simulink model "atrias_boom_nmSt_kinSw_v4"  (R2015a)
settings: Solver=ode23t  StartTime=0.0  StopTime=t_end  FixedStep=0.001  MaxStep=1e-3  RelTol=1e-3
InitFcn:
  | addpath('../common/')
  | colors
StartFcn:
  | tic
StopFcn:
  | %stopscript
values from neighbouring files (symbols this model uses):
  dt_a_dTrunk_boom = 5    [main_1_nmSt_kinSw.m]    (also in main_2_nmSt_kinSw_v2.m; main_3_nmSt_kinSw_v3.m; main_4_nmSt_kinSw_v4.m)
  dt_fade_boomCtrl = 2    [main_1_nmSt_kinSw.m]    (also in main_2_nmSt_kinSw_v2.m; main_3_nmSt_kinSw_v3.m; main_4_nmSt_kinSw_v4.m)
  initial_boom_yaw = 15*pi/180    (= 0.261799387799)    [main_2_nmSt_kinSw_v2.m]    (also in main_3_nmSt_kinSw_v3.m; main_4_nmSt_kinSw_v4.m)
  kd_boom_roll_Ctrl = 0    [main_1_nmSt_kinSw - Copy.m]    (also in main_1_nmSt_kinSw.m; main_2_nmSt_kinSw_v2.m; main_3_nmSt_kinSw_v3.m; main_4_nmSt_kinSw_v4.m)
  kd_boom_yaw_Ctrl = 0.1*kp_boom_yaw_Ctrl    (= 100000000)    [main_1_nmSt_kinSw - Copy.m]    (also in main_1_nmSt_kinSw.m = 1000000000; main_2_nmSt_kinSw_v2.m = 10000000; main_3_nmSt_kinSw_v3.m = 10000000; main_4_nmSt_kinSw_v4.m = 10000000)
  kd_motor = 0.90*2*sqrt(3.75*kp_motor)    [main_1_nmSt_kinSw - Copy.m]
  kinSw_alpha_start = 100*pi/180    (= 1.74532925199)    [main_1_nmSt_kinSw - Copy.m]    (also in main_1_nmSt_kinSw.m = 1.91986217719; main_2_nmSt_kinSw_v2.m = 1.83259571459; main_3_nmSt_kinSw_v3.m = 1.83259571459; main_4_nmSt_kinSw_v4.m = 1.83259571459)
  kinSw_alpha_tgt = 80*pi/180    (= 1.3962634016)    [main_1_nmSt_kinSw - Copy.m]    (also in main_1_nmSt_kinSw.m = 1.2217304764; main_2_nmSt_kinSw_v2.m = 1.2217304764; main_3_nmSt_kinSw_v3.m = 1.2217304764; main_4_nmSt_kinSw_v4.m = 1.2217304764)
  kinSw_t_start = 1.5    [main_1_nmSt_kinSw - Copy.m]    (also in main_1_nmSt_kinSw.m; main_2_nmSt_kinSw_v2.m = 0.5; main_3_nmSt_kinSw_v3.m = 0.5; main_4_nmSt_kinSw_v4.m = 0.5)
  kp_boom_roll_Ctrl = 0    [main_1_nmSt_kinSw - Copy.m]    (also in main_1_nmSt_kinSw.m; main_2_nmSt_kinSw_v2.m; main_3_nmSt_kinSw_v3.m; main_4_nmSt_kinSw_v4.m)
  kp_boom_yaw_Ctrl = 1e9    (= 1000000000)    [main_1_nmSt_kinSw - Copy.m]    (also in main_1_nmSt_kinSw.m = 10000000000; main_2_nmSt_kinSw_v2.m = 100000000; main_3_nmSt_kinSw_v3.m = 100000000; main_4_nmSt_kinSw_v4.m = 100000000)
  kp_motor = 3000    [main_1_nmSt_kinSw - Copy.m]
  max_back_bar_angle = 262.4*pi/180    (= 4.57974395723)    [main_1_nmSt_kinSw - Copy.m]
  max_front_bar_angle = 194.8*pi/180    (= 3.39990138288)    [main_1_nmSt_kinSw - Copy.m]
  min_back_bar_angle = 165.0*pi/180    (= 2.87979326579)    [main_1_nmSt_kinSw - Copy.m]
  min_front_bar_angle = 98.0*pi/180    (= 1.71042266695)    [main_1_nmSt_kinSw - Copy.m]
  poser_LLegAlp = (initial_l_leg_angle -pi/2)*180/pi    (= 105)    [main_2_nmSt_kinSw_v2.m]    (also in main_3_nmSt_kinSw_v3.m; main_4_nmSt_kinSw_v4.m)
  poser_LLegLen = initial_l_leg_length    (= 0.88)    [main_2_nmSt_kinSw_v2.m]    (also in main_3_nmSt_kinSw_v3.m; main_4_nmSt_kinSw_v4.m)
  poser_RLegAlp = (initial_r_leg_angle -pi/2)*180/pi    (= 75)    [main_2_nmSt_kinSw_v2.m]    (also in main_3_nmSt_kinSw_v3.m; main_4_nmSt_kinSw_v4.m)
  poser_RLegLen = initial_r_leg_length    (= 0.9)    [main_2_nmSt_kinSw_v2.m]    (also in main_3_nmSt_kinSw_v3.m; main_4_nmSt_kinSw_v4.m)
  tEnd_boomCtrl = t_end    (= 20)    [main_1_nmSt_kinSw - Copy.m]    (also in main_1_nmSt_kinSw.m = 3; main_2_nmSt_kinSw_v2.m = 7.5; main_3_nmSt_kinSw_v3.m = 7.5; main_4_nmSt_kinSw_v4.m = 7.5)
  tStart_boomCtrl = 1    [main_1_nmSt_kinSw - Copy.m]    (also in main_1_nmSt_kinSw.m = 0; main_2_nmSt_kinSw_v2.m = 0.5; main_3_nmSt_kinSw_v3.m = 0.5; main_4_nmSt_kinSw_v4.m = 0.5)
  tune_kinSw_alpha_start = kinSw_alpha_start*180/pi    (= 105)    [main_2_nmSt_kinSw_v2.m]    (also in main_3_nmSt_kinSw_v3.m; main_4_nmSt_kinSw_v4.m)
  tune_kinSw_alpha_tgt = kinSw_alpha_tgt*180/pi    (= 70)    [main_2_nmSt_kinSw_v2.m]    (also in main_3_nmSt_kinSw_v3.m; main_4_nmSt_kinSw_v4.m)
  tune_kinSw_gClr_tgt = kinSw_gClr    (= 0.15)    [main_4_nmSt_kinSw_v4.m]
  tune_kinSw_gH_tgt = kinSw_gH_tgt    (= -0.01)    [main_4_nmSt_kinSw_v4.m]
  tune_M1_G = St_FGain_VAS*FmaxVAS    [main_2_nmSt_kinSw_v2.m]    (also in main_3_nmSt_kinSw_v3.m; main_4_nmSt_kinSw_v4.m)
  tune_M3_0 = CtrlPar_theta0*180/pi    [main_2_nmSt_kinSw_v2.m]    (also in main_3_nmSt_kinSw_v3.m; main_4_nmSt_kinSw_v4.m)
  tune_M3_D = St_GainDTh_HFL    [main_2_nmSt_kinSw_v2.m]    (also in main_3_nmSt_kinSw_v3.m; main_4_nmSt_kinSw_v4.m)
  tune_M3_P = St_GainTh_HFL    [main_2_nmSt_kinSw_v2.m]    (also in main_3_nmSt_kinSw_v3.m; main_4_nmSt_kinSw_v4.m)
  tune_M4_G = 1    [main_3_nmSt_kinSw_v3.m]    (also in main_4_nmSt_kinSw_v4.m)
  v_dTrunk_boom = 1.3    [main_1_nmSt_kinSw.m]    (also in main_2_nmSt_kinSw_v2.m; main_3_nmSt_kinSw_v3.m; main_4_nmSt_kinSw_v4.m)
undefined symbols (not defined in the file or in its folder): A1_notch_f1, A2_notch_f1, A_lpf_dtau, A_lpf_velocity, ankle_stiffness, B1_lpf_dtau, B1_lpf_velocity, B1_notch_f1, B2_lpf_dtau, B2_lpf_velocity, B2_notch_f1, b_hmotor, b_leg_spring, b_rotor, base_color_d, boom_color_d, boom_mount_to_center_diagonal, breakaway_friction, c_jointstop, contactThr, coulomb_friction, d_com, delta_phi_max, delta_phi_max_buffer, delta_phi_max_dropoff, delta_phi_min, fblink_color_d, floor_color_d, FmaxBFSH, FmaxGLU, FmaxHAM, FmaxHFL, FmaxRF, FmaxVAS, foot_color_d, FPCtrlPar, friction_linear_zone, g, gain_nodes_sea_torque, HIP_MTR_MAX_CONT_TORQUE, HIP_MTR_MAX_TORQUE, hshaft_color_d, initial_boom_pitch, initial_boom_roll, initial_hip_roll, initial_winch_angle, j_motor, k_gn, k_gt, k_leg_spring, K_notch_f1, k_phi, k_sea, Kb_leg, kd_lateral, kd_shin_max, kd_shin_min, kd_splay_max, kd_splay_min, kd_thigh_max ... (+186)
libraries: sm_lib x210, nesl_utility x140, simulink x65, simulink_extras x32, fl_lib x16, mblibv1 x2, commnoisgen2 x1
(part 1 of 17)
settings Model: CovSFcnEnable=off  Creator=wmartin  LastModifiedBy=smsong
settings SolverCC: MaxOrder=2  MaxConsecutiveZCs=100  ZeroCrossAlgorithm=Adaptive  InsertRTBMode=Never (minimum delay)
settings DataIOCC: LimitDataPoints=off  SaveOutput=off  SignalLogging=off  DSMLogging=off  ReturnWorkspaceOutputs=on  OutputTimes=[0:1/30:45]
settings OptimizationCC: UseDivisionForNetSlopeComputation=UseDivisionForReciprocalsOfIntegersOnly  UseFloatMulNetSlope=on  EnhancedBackFolding=on  MemcpyThreshold=1024  EfficientFloat2IntCast=on  SimCompilerOptimization=on  AccelVerboseBuild=on
settings DebuggingCC: AlgebraicLoopMsg=none  UnconnectedInputMsg=none  UnconnectedOutputMsg=none  UnconnectedLineMsg=none  StateNameClashWarn=warning
settings ModelReferenceCC: UpdateModelReferenceTargets=IfOutOfDate
settings SFSimCC: SFSimOverflowDetection=off  SFSimEcho=off
settings RTWCC: BuildConfiguration=Faster Runs
settings GRTTargetCC: MatFileLogging=off  SupportNonFinite=off
settings ExplorerConfigSet: InternalSimMechanicsExplorerSettings="<ExplorerConfiguration><canonicalview>planar_xy</canonicalview><AnimationSetting><BasePlaybackSpeed>1.0</BasePlaybackSpeed><PlaybackSpeedFactor>0.125</PlaybackSpeedFactor></AnimationSetting><TilePanel><TileInfo><Tiles Columns=\"1\" Count=\"1\" Rows=\"1\"><Column Left=\"2\" Weight=\"1\"/><Column Left=\"1588\"/><Row Top=\"2\" Weight=\"1\"/><Row Top=\"952\"/><Tile Height=\"1\" Width=\"1\" X=\"0\" Y=\"0\"/></Tiles></TileInfo><SceneInfo><SceneViewer><BGColor><R>0.89803922176361084</R><G>0.89803922176361084</G><B>0.94901961088180542</B></BGColor><Camera><Position><X>0</X><Y>1.5296000242233276</Y><Z>-13.796973836269585</Z></Position><Center><X>0</X><Y>1.5296000242233276</Y><Z>0</Z></Center><Up><X>0</X><Y>1</Y><Z>0</Z></Up><Left>-3.2532129764556887</Left><Right>3.2532129764556887</Right><Bottom>-1.6375799953937531</Bottom><Top>1.6375799953937531</Top></Camera></SceneViewer></SceneInfo></TilePanel></ExplorerConfiguration>"

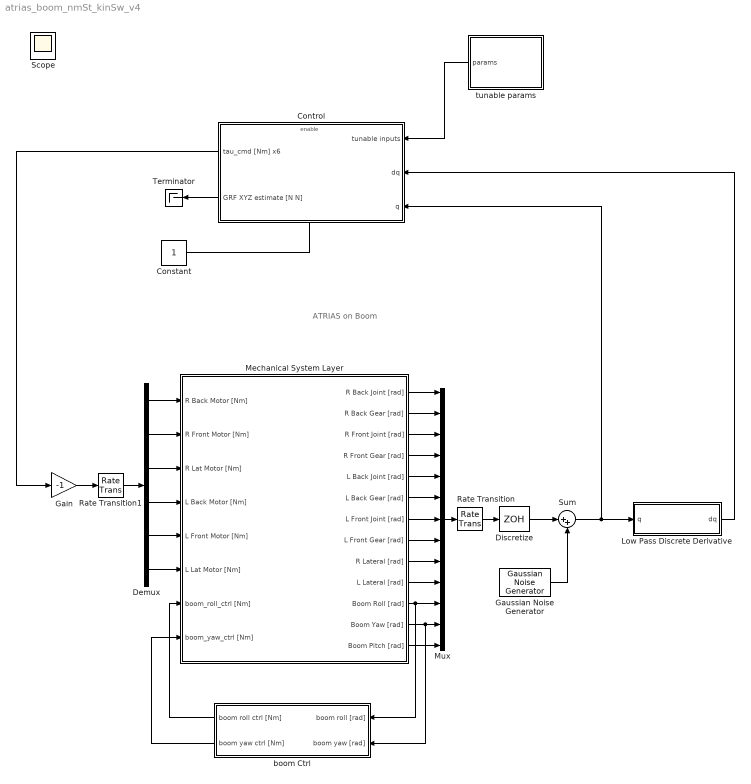
== system atrias_boom_nmSt_kinSw_v4 ==
  note: ATRIAS on Boom
  Constant : Constant
  Control : Subsystem
  Demux : Demux  Outputs=6
  Discretize : ZeroOrderHold  SampleTime=sample_time
  Gain : Gain  Gain=-1
  Gaussian Noise Generator : commnoisgen2/Gaussian Noise Generator  m=0  d=sensor_noise_variance  s=41  Ts=sample_time  frameBased=off  sampPerFrame=1  orient=off  outDataType=double
  Low Pass Discrete Derivative : Subsystem
  Mechanical System Layer : Subsystem
  Mux : Mux  Inputs=13
  Rate Transition : RateTransition  OutPortSampleTime=sample_time
  Rate Transition1 : RateTransition  OutPortSampleTime=sample_time
  Sum : Sum  Inputs=|++
  Terminator : Terminator
  boom Ctrl : Subsystem
  tunable params : Subsystem
  Scope : Scope
      settings: SaveName=ScopeData35
  wires:
  Mechanical System Layer/1(R Back Joint [rad]) -> Mux/1
  Mechanical System Layer/2(R Back Gear [rad]) -> Mux/2
  Mechanical System Layer/3(R Front Joint [rad]) -> Mux/3
  Mechanical System Layer/4(R Front Gear [rad]) -> Mux/4
  Mechanical System Layer/5(L Back Joint [rad]) -> Mux/5
  Mechanical System Layer/6(L Back Gear [rad]) -> Mux/6
  Mechanical System Layer/7(L Front Joint [rad]) -> Mux/7
  Mechanical System Layer/8(L Front Gear [rad]) -> Mux/8
  Mechanical System Layer/9(R Lateral [rad]) -> Mux/9
  Mechanical System Layer/10(L Lateral [rad]) -> Mux/10
  Mechanical System Layer/11(Boom Roll [rad]) -> boom Ctrl/1(boom roll [rad]), Mux/11
  Mechanical System Layer/12(Boom Yaw [rad]) -> boom Ctrl/2(boom yaw [rad]), Mux/12
  Mechanical System Layer/13(Boom Pitch [rad]) -> Mux/13
  Mux/1 -> Rate Transition/1
  Demux/1 -> Mechanical System Layer/1(R Back Motor [Nm])
  Demux/2 -> Mechanical System Layer/2(R Front Motor [Nm])
  Demux/3 -> Mechanical System Layer/3(R Lat Motor [Nm])
  Demux/4 -> Mechanical System Layer/4(L Back Motor [Nm])
  Demux/5 -> Mechanical System Layer/5(L Front Motor [Nm])
  Demux/6 -> Mechanical System Layer/6(L Lat Motor [Nm])
  Discretize/1 -> Sum/1
  Gaussian Noise Generator/1 -> Sum/2
  Rate Transition1/1 -> Demux/1
  Rate Transition/1 -> Discretize/1
  Low Pass Discrete Derivative/1(dq) -> Control/2(dq)
  Constant/1 -> Control/Enable
  Sum/1 -> Control/3(q), Low Pass Discrete Derivative/1(q)
  Control/2(GRF XYZ estimate [N N]) -> Terminator/1
  Control/1(tau_cmd [Nm] x6) -> Gain/1
  Gain/1 -> Rate Transition1/1
  boom Ctrl/2(boom yaw ctrl [Nm]) -> Mechanical System Layer/8(boom_yaw_ctrl [Nm])
  boom Ctrl/1(boom roll ctrl [Nm]) -> Mechanical System Layer/7(boom_roll_ctrl [Nm])
  tunable params/1(params) -> Control/1(tunable inputs)

== system atrias_boom_nmSt_kinSw_v4/Control ==
  tunable inputs : Inport
  dq : Inport  Port=2
  q : Inport  Port=3
  Enable : EnablePort  StatesWhenEnabling=reset  PropagateVarSize=During execution
  Actuator Control : Subsystem
  Behavior Control : Subsystem
  Tunable Control Parameters : Subsystem
  tau_cmd [Nm] x6 : Outport  InitialOutput=[0 0 0 0 0 0]
  GRF XYZ estimate [N N] : Outport  Port=2  InitialOutput=[0 0 0]
  wires:
  q/1 -> Actuator Control/4(q), Behavior Control/2(q [rad] x13)
  dq/1 -> Actuator Control/5(dq), Behavior Control/1(dq [rad/s] x13)
  Behavior Control/1(Motor Torque Command [Nm] x6) -> Actuator Control/1(Desired Torque [Nm] x6)
  Actuator Control/1(tau_cmd [Nm] x6) -> tau_cmd [Nm] x6/1
  Behavior Control/2(SEA Torque Velocity Command [Nm] x4) -> Actuator Control/2(Desired SEA Torque Velocity [Nm] x4)
  Behavior Control/3(Force / Position Control [1/0] x4) -> Actuator Control/3(Enable SEA Control [1/0] x4)
  Behavior Control/4(GRF XYZ estimates [N N N]) -> GRF XYZ estimate [N N]/1
  tunable inputs/1 -> Tunable Control Parameters/1(tunable inputs)

== system atrias_boom_nmSt_kinSw_v4/Low Pass Discrete Derivative ==
  q : Inport
  Gain1 : Gain  Gain=1/sample_time
  discrete difference : Subsystem
  two_pole_filter : DiscreteTransferFcn  Numerator=[A_lpf_velocity 0 0]  Denominator=[1 B1_lpf_velocity B2_lpf_velocity]  SampleTime=sample_time
  dq : Outport
  wires:
  q/1 -> discrete difference/1(in)
  two_pole_filter/1 -> dq/1
  Gain1/1 -> two_pole_filter/1
  discrete difference/1(out) -> Gain1/1

== system atrias_boom_nmSt_kinSw_v4/Mechanical System Layer ==
  R Back Motor [Nm] : Inport
  R Front Motor [Nm] : Inport  Port=2
  R Lat Motor [Nm] : Inport  Port=3
  L Back Motor [Nm] : Inport  Port=4
  L Front Motor [Nm] : Inport  Port=5
  L Lat Motor [Nm] : Inport  Port=6
  boom_roll_ctrl [Nm] : Inport  Port=7
  boom_yaw_ctrl [Nm] : Inport  Port=8
  Boom : Subsystem
      mask Display: image('../images/boom.png');
  Boom Base : Subsystem
      mask Display: image('../images/boom_base.png');
  Floor : Subsystem
  Floor Frame : sm_lib/Frames and Transforms/Rigid Transform  TranslationMethod=Cartesian  TranslationLengthUnit=m  TranslationStandardAxis=+Z  TranslationStandardOffset=0  TranslationCartesianOffset=[0 -0.03 0]  TranslationROffset=0  TranslationROffsetUnits=m  TranslationZOffset=0  TranslationZOffsetUnits=m  TranslationThetaOffset=0  TranslationThetaOffsetUnits=deg  RotationMethod=AlignedAxes  RotationAngleUnits=deg  RotationStandardAxis=+Z  RotationAngle=0  RotationArbitraryAxis=[0 0 1]  FollAlignAxisA=+Z  BaseAlignAxisA=+Y  FollAlignAxisB=+X  BaseAlignAxisB=+X  RotationMatrix=[1 0 0; 0 1 0; 0 0 1]  BlockFunction=simmechanics.library.frames_transforms.rigid_transform
  Ground : Subsystem
  Ground Contact Models : Subsystem
  L Hip Shaft : Subsystem
      mask Display: image(flipdim(imread('../images/hipshaft.JPG'),2));
  L Leg : Subsystem
      mask Display: image('../images/leg.JPG');
  Left Foot : Subsystem
      mask Display: image('../images/foot.png');
  Left Hip Roll Joint : Subsystem
  Pitch Joint : Subsystem
  R Hip Shaft : Subsystem
      mask Display: image('../images/hipshaft.JPG');
  R Leg : Subsystem
      mask Display: image('../images/leg.JPG');
  Right Foot : Subsystem
      mask Display: image('../images/foot.png');
  Right Hip Roll Joint : Subsystem
  Torso : Subsystem
      mask Display: image('../images/torso.png');
  Winch : Subsystem
  Yaw Joint : Subsystem
  Yaw Shaft : Subsystem
      mask Display: image('../images/boom_yaw_shaft.png');
  R Back Joint [rad] : Outport
  R Back Gear [rad] : Outport  Port=2
  R Front Joint [rad] : Outport  Port=3
  R Front Gear [rad] : Outport  Port=4
  L Back Joint [rad] : Outport  Port=5
  L Back Gear [rad] : Outport  Port=6
  L Front Joint [rad] : Outport  Port=7
  L Front Gear [rad] : Outport  Port=8
  R Lateral [rad] : Outport  Port=9
  L Lateral [rad] : Outport  Port=10
  Boom Roll [rad] : Outport  Port=11
  Boom Yaw [rad] : Outport  Port=12
  Boom Pitch [rad] : Outport  Port=13
  tag scope: qYaw=global
  wires:
  L Leg/1(Shin Joint [rad]) -> L Back Joint [rad]/1
  R Back Motor [Nm]/1 -> R Leg/1(Shin Motor [Nm])
  L Back Motor [Nm]/1 -> L Leg/1(Shin Motor [Nm])
  Right Hip Roll Joint/1(Hip Roll [rad]) -> R Lateral [rad]/1
  L Leg/3(Thigh Joint [rad]) -> L Front Joint [rad]/1
  Winch/1(Boom Roll [rad]) -> Boom Roll [rad]/1
  Left Hip Roll Joint/1(Hip Roll [rad]) -> L Lateral [rad]/1
  L Leg/4(Thigh Gear [rad]) -> L Front Gear [rad]/1
  R Leg/1(Shin Joint [rad]) -> R Back Joint [rad]/1
  R Leg/2(Shin Gear [rad]) -> R Back Gear [rad]/1
  L Leg/2(Shin Gear [rad]) -> L Back Gear [rad]/1
  R Leg/4(Thigh Gear [rad]) -> R Front Gear [rad]/1
  L Front Motor [Nm]/1 -> L Leg/2("Thigh Motor [Nm]  ")
  R Lat Motor [Nm]/1 -> Right Hip Roll Joint/1(Hip Motor [Nm])
  R Front Motor [Nm]/1 -> R Leg/2("Thigh Motor [Nm]  ")
  L Lat Motor [Nm]/1 -> Left Hip Roll Joint/1(Hip Motor [Nm])
  R Leg/3(Thigh Joint [rad]) -> R Front Joint [rad]/1
  Pitch Joint/1(Pitch [rad]) -> Boom Pitch [rad]/1
  Yaw Joint/1(Yaw [rad]) -> [qYaw], Boom Yaw [rad]/1
  boom_roll_ctrl [Nm]/1 -> Winch/1(boom_roll_ctrl [Nm])
  boom_yaw_ctrl [Nm]/1 -> Yaw Joint/1(boom_yaw_ctrl [Nm])
  connections:
  Torso/LConn1 -- Left Hip Roll Joint/RConn1
  Right Hip Roll Joint/RConn1 -- R Hip Shaft/RConn1
  Winch/RConn2 -- Yaw Shaft/RConn1
  Left Hip Roll Joint/LConn1 -- L Hip Shaft/LConn1
  Right Foot/LConn1 -- R Leg/LConn1
  R Leg/RConn1 -- R Hip Shaft/LConn1
  Torso/LConn2 -- Right Hip Roll Joint/LConn1
  L Leg/LConn1 -- L Hip Shaft/RConn1
  Left Foot/LConn1 -- L Leg/RConn1
  Pitch Joint/LConn1 -- Torso/RConn1
  Floor Frame/RConn1 -- Floor/LConn1
  Floor Frame/LConn1 -- Ground/RConn1 -- Boom Base/LConn1
  Boom/LConn1 -- Winch/RConn1
  Yaw Shaft/LConn1 -- Yaw Joint/RConn1
  Yaw Joint/LConn1 -- Boom Base/RConn1
  Pitch Joint/RConn1 -- Boom/RConn1
  Left Foot/RConn1 -- Ground Contact Models/RConn1
  Left Foot/RConn2 -- Ground Contact Models/RConn2
  Right Foot/RConn1 -- Ground Contact Models/RConn3
  Right Foot/RConn2 -- Ground Contact Models/RConn4

== system atrias_boom_nmSt_kinSw_v4/boom Ctrl ==
  boom roll [rad] : Inport
  boom yaw [rad] : Inport  Port=2
  Clock : Clock
  Constant1 : Constant  Value=tStart_boomCtrl
  Constant2 : Constant  Value=tEnd_boomCtrl
  Logical Operator : Logic  AllPortsSameDT=off  OutDataTypeStr=boolean
  Relational Operator : RelationalOperator  OutDataTypeStr=boolean
  Relational Operator1 : RelationalOperator  Operator=<=  OutDataTypeStr=boolean
  boom Ctrl : Subsystem
  boom roll ctrl [Nm] : Outport
  boom yaw ctrl [Nm] : Outport  Port=2
  wires:
  Relational Operator/1 -> Logical Operator/1
  Relational Operator1/1 -> Logical Operator/2
  Constant2/1 -> Relational Operator1/2
  boom yaw [rad]/1 -> boom Ctrl/2(Boom Yaw [rad])
  Constant1/1 -> Relational Operator/2
  boom roll [rad]/1 -> boom Ctrl/1(Boom Roll [rad])
  Logical Operator/1 -> boom Ctrl/Enable
  Clock/1 -> Relational Operator1/1, Relational Operator/1
  boom Ctrl/1(boom_roll_ctrl [Nm]) -> boom roll ctrl [Nm]/1  "roll"
  boom Ctrl/2(boom_yaw_ctrl [Nm]) -> boom yaw ctrl [Nm]/1  "yaw"

== system atrias_boom_nmSt_kinSw_v4/tunable params ==
  note: do not forget to set the params of the low pass filters!!
  Constant1 : Constant  Value=tune_M4_G
  Constant11 : Constant  Value=tune_M1_G
  Constant12 : Constant  Value=tune_M3_0
  Constant18 : Constant  Value=tune_M3_D
  Constant20 : Constant  Value=tune_M3_P
  Constant28 : Constant  Value=poser_RLegLen
  Constant29 : Constant  Value=poser_RLegAlp
  Constant30 : Constant  Value=poser_LLegLen
  Constant31 : Constant  Value=poser_LLegAlp
  Constant36 : Constant  Value=tune_kinSw_alpha_start
  Constant37 : Constant  Value=tune_kinSw_alpha_tgt
  Constant38 : Constant  Value=tune_kinSw_gH_tgt
  Constant39 : Constant  Value=tune_kinSw_gClr_tgt
  Mux2 : Mux  Inputs=13
  low pass filter : simulink_extras/Additional Linear/Transfer Fcn (with initial outputs)  N=[1]  D="[.5  1]"  Y0=tune_M1_G  U0=tune_M1_G
      settings: AttributesFormatString=pre-activation: %<Y0>
  low pass filter1 : simulink_extras/Additional Linear/Transfer Fcn (with initial outputs)  N=[1]  D="[.5  1]"  Y0=tune_M3_0  U0=tune_M3_0
      settings: AttributesFormatString=pre-activation: %<Y0>
  low pass filter10 : simulink_extras/Additional Linear/Transfer Fcn (with initial outputs)  N=[1]  D="[.5  1]"  Y0=poser_LLegLen  U0=poser_LLegLen
      settings: AttributesFormatString=pre-activation: %<Y0>
  low pass filter11 : simulink_extras/Additional Linear/Transfer Fcn (with initial outputs)  N=[1]  D="[.5  1]"  Y0=poser_LLegAlp  U0=poser_LLegAlp
      settings: AttributesFormatString=pre-activation: %<Y0>
  low pass filter12 : simulink_extras/Additional Linear/Transfer Fcn (with initial outputs)  N=[1]  D="[.5  1]"  Y0=tune_M4_G  U0=tune_M4_G
      settings: AttributesFormatString=pre-activation: %<Y0>
  low pass filter2 : simulink_extras/Additional Linear/Transfer Fcn (with initial outputs)  N=[1]  D="[.5  1]"  Y0=tune_M3_P  U0=tune_M3_P
      settings: AttributesFormatString=pre-activation: %<Y0>
  low pass filter3 : simulink_extras/Additional Linear/Transfer Fcn (with initial outputs)  N=[1]  D="[.5  1]"  Y0=tune_M3_D  U0=tune_M3_D
      settings: AttributesFormatString=pre-activation: %<Y0>
  low pass filter4 : simulink_extras/Additional Linear/Transfer Fcn (with initial outputs)  N=[1]  D="[.5  1]"  Y0=tune_kinSw_alpha_start  U0=tune_kinSw_alpha_start
      settings: AttributesFormatString=pre-activation: %<Y0>
  low pass filter5 : simulink_extras/Additional Linear/Transfer Fcn (with initial outputs)  N=[1]  D="[.5  1]"  Y0=tune_kinSw_alpha_tgt  U0=tune_kinSw_alpha_tgt
      settings: AttributesFormatString=pre-activation: %<Y0>
  low pass filter6 : simulink_extras/Additional Linear/Transfer Fcn (with initial outputs)  N=[1]  D="[.5  1]"  Y0=tune_kinSw_gH_tgt  U0=tune_kinSw_gH_tgt
      settings: AttributesFormatString=pre-activation: %<Y0>
  low pass filter7 : simulink_extras/Additional Linear/Transfer Fcn (with initial outputs)  N=[1]  D="[.5  1]"  Y0=tune_kinSw_gClr_tgt  U0=tune_kinSw_gClr_tgt
      settings: AttributesFormatString=pre-activation: %<Y0>
  low pass filter8 : simulink_extras/Additional Linear/Transfer Fcn (with initial outputs)  N=[1]  D="[.5  1]"  Y0=poser_RLegLen  U0=poser_RLegLen
      settings: AttributesFormatString=pre-activation: %<Y0>
  low pass filter9 : simulink_extras/Additional Linear/Transfer Fcn (with initial outputs)  N=[1]  D="[.5  1]"  Y0=poser_RLegAlp  U0=poser_RLegAlp
      settings: AttributesFormatString=pre-activation: %<Y0>
  params : Outport
  wires:
  Mux2/1 -> params/1
  Constant18/1 -> low pass filter3/1
  Constant11/1 -> low pass filter/1
  Constant36/1 -> low pass filter4/1
  Constant37/1 -> low pass filter5/1
  Constant12/1 -> low pass filter1/1
  Constant38/1 -> low pass filter6/1
  Constant39/1 -> low pass filter7/1
  Constant20/1 -> low pass filter2/1
  low pass filter/1 -> Mux2/1
  low pass filter1/1 -> Mux2/2
  low pass filter2/1 -> Mux2/3
  low pass filter3/1 -> Mux2/4
  low pass filter4/1 -> Mux2/6
  low pass filter5/1 -> Mux2/7
  low pass filter6/1 -> Mux2/8
  low pass filter7/1 -> Mux2/9
  Constant28/1 -> low pass filter8/1
  low pass filter8/1 -> Mux2/10
  Constant29/1 -> low pass filter9/1
  low pass filter9/1 -> Mux2/11
  Constant30/1 -> low pass filter10/1
  low pass filter10/1 -> Mux2/12
  Constant31/1 -> low pass filter11/1
  low pass filter11/1 -> Mux2/13
  Constant1/1 -> low pass filter12/1
  low pass filter12/1 -> Mux2/5

== system atrias_boom_nmSt_kinSw_v4/Control/Actuator Control ==
  note: Order:
      | backR
      | frontR
      | backL
      | frontL
  note: Motor Order:
      |
      | backR
      | frontR
      | latR
      | backL
      | frontL
      | latL
  Desired Torque [Nm] x6 : Inport  OutDataTypeStr=double  PortDimensions=6  SampleTime=sample_time
  Desired SEA Torque Velocity [Nm] x4 : Inport  Port=2  OutDataTypeStr=double  PortDimensions=4  SampleTime=sample_time
  Enable SEA Control [1/0] x4 : Inport  Port=3  OutDataTypeStr=boolean  PortDimensions=4  SampleTime=sample_time
  q : Inport  Port=4  OutDataTypeStr=double  PortDimensions=13  SampleTime=sample_time
  dq : Inport  Port=5  OutDataTypeStr=double  PortDimensions=13  SampleTime=sample_time
  Activate SEA Control : Subsystem
  Antiresonance Compensation : Subsystem
  Hip Motor Efficiency Compensation : Gain  Gain=1/lateral_motor_efficiency
  Leg Motor Efficiency Compensation : Gain  Gain=1/sagittal_motor_efficiency
  Mux{1..2,4..5} (4 alike) : Mux
  Mux3 : Mux  Inputs=2
  SEA Control Toggle : Subsystem
  SEA Controller (Torque) : Subsystem
  Selector12 : Selector  InputPortWidth=13  Indices=[5 6]
  Selector13 : Selector  InputPortWidth=13  Indices=[7 8]
  Selector15 : Selector  InputPortWidth=13  Indices=[1 2]
  Selector16 : Selector  InputPortWidth=13  Indices=[3 4]
  Selector{17..20,25..28} (8 alike) : Selector  InputPortWidth=2  Indices=[1]
  Selector2 : Selector  InputPortWidth=13  Indices=[5 6]
  Selector{21..24,29..32} (8 alike) : Selector  InputPortWidth=2  Indices=[2]
  Selector3 : Selector  InputPortWidth=6  Indices=[3 6]
  Selector33 : Selector  InputPortWidth=6  Indices=[1 2 4 5]
  Selector4 : Selector  InputPortWidth=13  Indices=[7 8]
  Selector6 : Selector  InputPortWidth=13  Indices=[1 2]
  Selector7 : Selector  InputPortWidth=13  Indices=[3 4]
  Selector8 : Selector  InputPortWidth=6  Indices=[1 2 5 3 4 6]
  Selector9 : Selector  InputPortWidth=6  Indices=[1 2 4 5]
  Terminator1 : Terminator
  Torque Limiter (outside) 1 : Saturate  UpperLimit=max_sagittal_unloaded_torque  LowerLimit=-max_sagittal_unloaded_torque
      settings: AttributesFormatString=Hi: %<UpperLimit>\nLo: %<LowerLimit>
  tau_desired_signals : Gain  Description=xPCTag(1)=tau_cmd_signal;
  tau_cmd [Nm] x6 : Outport  OutDataTypeStr=double  PortDimensions=6  SampleTime=0  InitialOutput=[0 0 0 0 0 0]
  wires:
  Selector3/1 -> Hip Motor Efficiency Compensation/1
  [dqFrontL] -> Selector32/1
  Selector29/1 -> Mux5/1
  Selector18/1 -> Mux1/2
  Selector19/1 -> Mux1/3
  Selector2/1 -> [qBackL]
  Selector15/1 -> [dqBackR]
  dq/1 -> Selector13/1, Selector15/1, Selector16/1, Selector12/1
  tau_desired_signals/1 -> Terminator1/1
  Selector7/1 -> [qFrontR]
  Torque Limiter (outside) 1/1 -> Activate SEA Control/3(Torque Signal [Nm] x4), SEA Control Toggle/3(tau_cmd)
  Desired Torque [Nm] x6/1 -> Selector33/1, Selector9/1, Selector3/1, tau_desired_signals/1
  Selector8/1 -> tau_cmd [Nm] x6/1
  Selector6/1 -> [qBackR]
  SEA Controller (Torque)/1(tau_cmd sagittal [Nm] x4) -> Activate SEA Control/1(SEA Control Signal [Nm] x4)
  SEA Controller (Torque)/2(tau_measured [Nm] x4) -> SEA Control Toggle/2(tau_measured)
  Activate SEA Control/1(Torque Command [Nm] x4) -> Leg Motor Efficiency Compensation/1
  q/1 -> Selector2/1, Selector7/1, Selector6/1, Selector4/1
  Selector16/1 -> [dqFrontR]
  Selector4/1 -> [qFrontL]
  Selector9/1 -> Antiresonance Compensation/1(Torque)
  [qBackL] -> Selector23/1
  Selector26/1 -> Mux4/2
  Selector30/1 -> Mux5/2
  Mux5/1 -> SEA Controller (Torque)/6(dphi_gear [rad/s] x4)
  Leg Motor Efficiency Compensation/1 -> Mux3/1
  Selector24/1 -> Mux2/4
  [qFrontR] -> Selector18/1
  [qFrontL] -> Selector20/1
  [qBackR] -> Selector21/1
  Antiresonance Compensation/1(Filtered Torque) -> Torque Limiter (outside) 1/1
  Selector13/1 -> [dqFrontL]
  Selector23/1 -> Mux2/3
  Mux1/1 -> SEA Controller (Torque)/1(phi_load [rad] x4)
  [dqFrontL] -> Selector28/1
  Desired SEA Torque Velocity [Nm] x4/1 -> SEA Controller (Torque)/4(dtau_des sagittal [Nm] x4)
  Selector25/1 -> Mux4/1
  Selector31/1 -> Mux5/3
  [dqBackL] -> Selector31/1
  Hip Motor Efficiency Compensation/1 -> Mux3/2
  Selector28/1 -> Mux4/4
  [qFrontL] -> Selector24/1
  Selector22/1 -> Mux2/2
  [dqFrontR] -> Selector30/1
  Selector32/1 -> Mux5/4
  Mux4/1 -> SEA Controller (Torque)/5(dphi_load [rad/s] x4)
  Mux3/1 -> Selector8/1
  [dqBackR] -> Selector29/1
  Selector27/1 -> Mux4/3
  [qFrontR] -> Selector22/1
  Selector21/1 -> Mux2/1
  [dqBackL] -> Selector27/1
  [dqBackR] -> Selector25/1
  Selector20/1 -> Mux1/4
  Selector17/1 -> Mux1/1
  [qBackR] -> Selector17/1
  [qBackL] -> Selector19/1
  Selector12/1 -> [dqBackL]
  Mux2/1 -> SEA Controller (Torque)/2(phi_gear [rad] x4)
  SEA Control Toggle/1(SEA Control on/off [1/0]) -> Activate SEA Control/2("SEA on/off [1/0] x4 ")
  Selector33/1 -> SEA Controller (Torque)/3(tau_des sagittal [Nm] x4)
  Enable SEA Control [1/0] x4/1 -> SEA Control Toggle/1(enable)
  [dqFrontR] -> Selector26/1

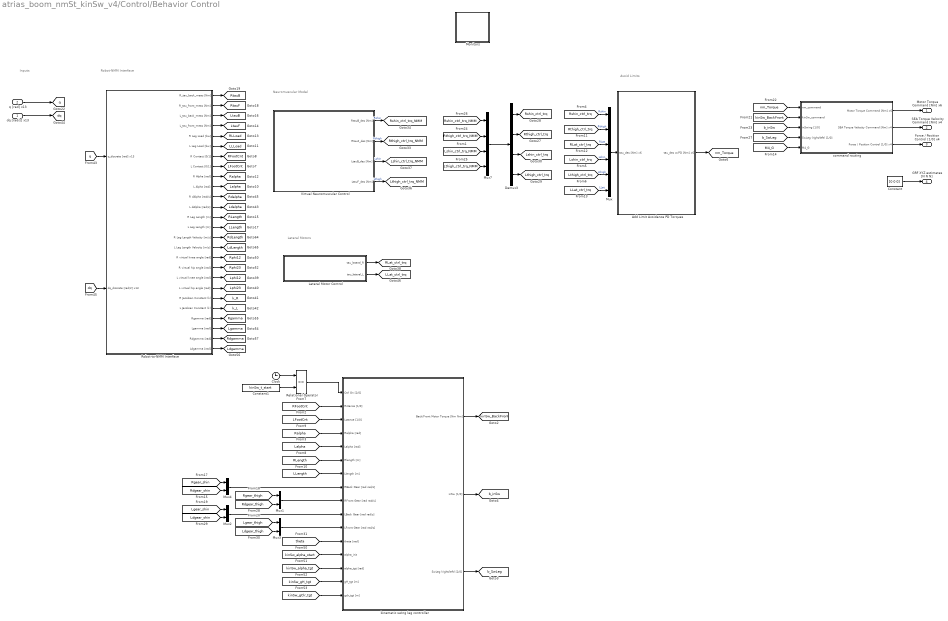
== system atrias_boom_nmSt_kinSw_v4/Control/Behavior Control ==
  note: Robot-NMM Interface
  note: Inputs
  note: Neuromuscular Model
  note: Avoid Limits
  note: Lateral Motors
  dq [rad/s] x13 : Inport
  q [rad] x13 : Inport  Port=2
  Add Limit Avoidance PD Torques : Subsystem
  Clock : Clock
  Constant : Constant  Value=[0 0 0]
  Constant1 : Constant  Value=kinSw_t_start
  Demux3 : Demux
  Lateral Motor Control : Subsystem
  Monitors : Subsystem
  Mux : Mux  Inputs=6
  Mux{1..4} (4 alike) : Mux  Inputs=2
  Mux7 : Mux
  Relational Operator : RelationalOperator
  Robot-to-NMM Interface : Subsystem
  Virtual Neuromuscular Control : Subsystem  SystemSampleTime=sample_time
  command routing : Subsystem
  kinematic swing leg controller : Subsystem
  Motor Torque Command [Nm] x6 : Outport  OutputWhenDisabled=reset  InitialOutput=[0 0 0 0 0 0]
  SEA Torque Velocity Command [Nm] x4 : Outport  Port=2  OutputWhenDisabled=reset  InitialOutput=[0 0 0 0 0 0]
  Force / Position Control [1/0] x4 : Outport  Port=3  OutputWhenDisabled=reset  InitialOutput=[0 0 0 0 0 0]
  GRF XYZ estimates [N N N] : Outport  Port=4  OutputWhenDisabled=reset  InitialOutput=[0 0 0 0 0 0]
  tag scope: LFootCnt=global, LLLoad=global, LLat_ctrl_trq=global, LLength=global, Lalpha=global, LdLength=global, Ldalpha=global, Ldgamma=global, Lgamma=global, Lphi12=global, Lphi23=global, Lshin_ctrl_trq=global, Lshin_ctrl_trq_NMM=global, LtauB=global, LtauF=global, Lthigh_ctrl_trq=global, Lthigh_ctrl_trq_NMM=global, RFootCnt=global, RLLoad=global, RLat_ctrl_trq=global, RLength=global, Ralpha=global, RdLength=global, Rdalpha=global, Rdgamma=global, Rgamma=global, Rphi12=global, Rphi23=global, Rshin_ctrl_trq=global, Rshin_ctrl_trq_NMM=global, RtauB=global, RtauF=global, Rthigh_ctrl_trq=global, Rthigh_ctrl_trq_NMM=global, b_SwLeg=global, b_inSw=global, dq=global, k_L=global, k_R=global, kinSw_BackFront=global, nm_Torque=global, q=global
  wires:
  [q] -> Robot-to-NMM Interface/1(q_discrete [rad] x13)
  [dq] -> Robot-to-NMM Interface/2(dq_discrete [rad/2] x13)
  Robot-to-NMM Interface/6(L Leg Load [bw]) -> [LLLoad]
  Robot-to-NMM Interface/5(R Leg Load [bw]) -> [RLLoad]
  Robot-to-NMM Interface/10(L Alpha [rad]) -> [Lalpha]
  Robot-to-NMM Interface/9(R Alpha [rad]) -> [Ralpha]
  Robot-to-NMM Interface/14(L Leg Length [m]) -> [LLength]
  Robot-to-NMM Interface/13(R Leg Length [m]) -> [RLength]
  Robot-to-NMM Interface/7(R Contact [0/1]) -> [RFootCnt]
  Robot-to-NMM Interface/8(L Contact [0/1]) -> [LFootCnt]
  Robot-to-NMM Interface/4(L_tau_front_meas [Nm]) -> [LtauF]
  Robot-to-NMM Interface/3(L_tau_back_meas [Nm]) -> [LtauB]
  Robot-to-NMM Interface/2(R_tau_front_meas [Nm]) -> [RtauF]
  Robot-to-NMM Interface/1(R_tau_back_meas [Nm]) -> [RtauB]
  Robot-to-NMM Interface/17(R virtual knee angle [rad]) -> [Rphi12]
  Robot-to-NMM Interface/18(R virtual hip angle [rad]) -> [Rphi23]
  Robot-to-NMM Interface/19(L virtual knee angle [rad]) -> [Lphi12]
  Robot-to-NMM Interface/20(L virtual hip angle [rad]) -> [Lphi23]
  Robot-to-NMM Interface/22(L Jacobian Constant (k)) -> [k_L]
  Robot-to-NMM Interface/21(R Jacobian Constant (k)) -> [k_R]
  Robot-to-NMM Interface/11(R dAlpha [rad/s]) -> [Rdalpha]
  Robot-to-NMM Interface/12(L dAlpha [rad/s]) -> [Ldalpha]
  Robot-to-NMM Interface/23(Rgamma [rad]) -> [Rgamma]
  Robot-to-NMM Interface/24(Lgamma [rad]) -> [Lgamma]
  Robot-to-NMM Interface/25(Rdgamma [rad]) -> [Rdgamma]
  Robot-to-NMM Interface/26(Ldgamma [rad]) -> [Ldgamma]
  Robot-to-NMM Interface/15(R Leg Length Velocity [m/s]) -> [RdLength]
  Robot-to-NMM Interface/16(L Leg Length Velocity [m/s]) -> [LdLength]
  Virtual Neuromuscular Control/1(RtauB_des [Nm]) -> [Rshin_ctrl_trq_NMM]  "Rshin"
  Virtual Neuromuscular Control/2(RtauF_des [Nm]) -> [Rthigh_ctrl_trq_NMM]  "Rthigh"
  Virtual Neuromuscular Control/3(LtauB_des [Nm]) -> [Lshin_ctrl_trq_NMM]  "Lshin"
  [Rshin_ctrl_trq_NMM] -> Mux7/1
  [Rthigh_ctrl_trq_NMM] -> Mux7/2
  [Lshin_ctrl_trq_NMM] -> Mux7/3
  [Lthigh_ctrl_trq_NMM] -> Mux7/4
  Demux3/4 -> [Lthigh_ctrl_trq]
  Demux3/3 -> [Lshin_ctrl_trq]
  Demux3/2 -> [Rthigh_ctrl_trq]
  Demux3/1 -> [Rshin_ctrl_trq]
  [Rshin_ctrl_trq] -> Mux/1  "Rshin"
  [Rthigh_ctrl_trq] -> Mux/2  "Rthigh"
  [RLat_ctrl_trq] -> Mux/3  "RLat"
  [Lshin_ctrl_trq] -> Mux/4  "Lshin"
  [Lthigh_ctrl_trq] -> Mux/5  "Lthigh"
  [LLat_ctrl_trq] -> Mux/6  "LLat"
  Mux/1 -> Add Limit Avoidance PD Torques/1(tau_des [Nm] x6)
  Lateral Motor Control/2(tau_lateral_L) -> [LLat_ctrl_trq]
  Lateral Motor Control/1(tau_lateral_R) -> [RLat_ctrl_trq]
  Constant/1 -> GRF XYZ estimates [N N N]/1
  q [rad] x13/1 -> [q]
  dq [rad/s] x13/1 -> [dq]
  Virtual Neuromuscular Control/4(LtauF_des [Nm]) -> [Lthigh_ctrl_trq_NMM]  "Lthigh"
  Mux7/1 -> Demux3/1
  [Ralpha] -> kinematic swing leg controller/4(Ralpha [rad])
  [Lalpha] -> kinematic swing leg controller/5(Lalpha [rad])
  [RFootCnt] -> kinematic swing leg controller/2(Rstance [1/0])
  [LFootCnt] -> kinematic swing leg controller/3(Lstance [1/0])
  [RLength] -> kinematic swing leg controller/6(Rlength [m])
  [LLength] -> kinematic swing leg controller/7(Llength [m])
  kinematic swing leg controller/1(Back/Front Motor Torque [Nm Nm]) -> [kinSw_BackFront]
  kinematic swing leg controller/3(SwLeg (right/left) [1/0]) -> [b_SwLeg]
  kinematic swing leg controller/2(inSw [1/0]) -> [b_inSw]
  Add Limit Avoidance PD Torques/1(tau_des w/PD [Nm] x6) -> [nm_Torque]
  [kinSw_BackFront] -> command routing/2(kinSw_command)
  [nm_Torque] -> command routing/1(nm_command)
  [b_inSw] -> command routing/3(inSwing [1/0])
  [b_SwLeg] -> command routing/4(SwLeg (right/left) [1/0])
  command routing/3(Force / Position Control [1/0] x4) -> Force / Position Control [1/0] x4/1
  [Rdgear_shin] -> Mux4/2
  [Rdgear_thigh] -> Mux1/2
  [Rgear_shin] -> Mux4/1
  [Rgear_thigh] -> Mux1/1
  [Lgear_shin] -> Mux2/1
  [Ldgear_shin] -> Mux2/2
  [Lgear_thigh] -> Mux3/1
  [Ldgear_thigh] -> Mux3/2
  Mux1/1 -> kinematic swing leg controller/9(RFront Gear [rad rad/s])
  Mux4/1 -> kinematic swing leg controller/8(RBack Gear [rad rad/s])
  Mux2/1 -> kinematic swing leg controller/10(LBack Gear [rad rad/s])
  Mux3/1 -> kinematic swing leg controller/11(LFront Gear [rad rad/s])
  command routing/1(Motor Torque Command [Nm] x6) -> Motor Torque Command [Nm] x6/1
  command routing/2(SEA Torque Velocity Command [Nm] x4) -> SEA Torque Velocity Command [Nm] x4/1
  Clock/1 -> Relational Operator/1
  Constant1/1 -> Relational Operator/2
  Relational Operator/1 -> kinematic swing leg controller/1(Ctrl On [1/0])
  [theta] -> kinematic swing leg controller/12(theta [rad])
  [kinSw_alpha_start] -> kinematic swing leg controller/13(alpha_init)
  [kinSw_alpha_tgt] -> kinematic swing leg controller/14(alpha_tgt [rad])
  [M4_G] -> command routing/5(M4_G)
  [kinSw_gH_tgt] -> kinematic swing leg controller/15(gH_tgt [m])
  [kinSw_gClr_tgt] -> kinematic swing leg controller/16(gclr_tgt [m])

== system atrias_boom_nmSt_kinSw_v4/Control/Tunable Control Parameters ==
  note: main controller
  note: intial poser
  tunable inputs : Inport
  Constant1 : Constant  Value=St_PreSHFL
  Constant10 : Constant  Value=TrCtrlPar
  Constant13 : Constant  Value=St_loffBFSH_VAS
  Constant14 : Constant  Value=St_LGainBFSH_VAS
  Constant15 : Constant  Value=St_loffBFSH
  Constant16 : Constant  Value=St_LGain_BFSH
  Constant17 : Constant  Value=St_SGainCGLU_HFL
  Constant19 : Constant  Value=St_SGainCHAM_HFL
  Constant2 : Constant  Value=LLCtrlPar
  Constant21 : Constant  Value=St_SGainGLU_HAM
  Constant22 : Constant  Value=St_SGainCHFL_GLU
  Constant23 : Constant  Value=St_SGainCRF_GLU
  Constant24 : Constant  Value=pi/2
  Constant3 : Constant  Value=St_PreSGLU
  Constant4 : Constant  Value=St_PreSHAM
  Constant5 : Constant  Value=St_PreSRF
  Constant6 : Constant  Value=FPCtrlPar
  Constant7 : Constant  Value=St_PreSVAS
  Constant8 : Constant  Value=St_PreSBFSH
  Constant9 : Constant  Value=SwCtrlPar
  Demux1 : Demux  Outputs=13
  Gain : Gain  Gain=1/FmaxVAS
  Gain{1..5} (5 alike) : Gain  Gain=pi/180
  Mux : Mux  Inputs=21
  Sum : Sum  Inputs=|++
  Sum1 : Sum  Inputs=|++
  tag scope: FPCtrlPar=global, LLCtrlPar=global, M4_G=global, StCtrlPar=global, SwCtrlPar=global, TrCtrlPar=global, kinSw_alpha_start=global, kinSw_alpha_tgt=global, kinSw_gClr_tgt=global, kinSw_gH_tgt=global, poser_LLegAng=global, poser_LLegLen=global, poser_RLegAng=global, poser_RLegLen=global, theta0=global
  wires:
  Constant6/1 -> [FPCtrlPar]
  Constant10/1 -> [TrCtrlPar]
  Constant9/1 -> [SwCtrlPar]
  Constant2/1 -> [LLCtrlPar]
  [tune_M3_0] -> Gain1/1
  [tune_M1_G] -> Gain/1
  Mux/1 -> [StCtrlPar]
  Gain1/1 -> [theta0]
  [poser_RLegLen] -> [poser_RLegLen]
  Sum/1 -> [poser_RLegAng]
  [poser_LLegLen] -> [poser_LLegLen]
  Sum1/1 -> [poser_LLegAng]
  [tune_kinSw_alpha_start] -> Gain4/1
  [tune_kinSw_alpha_tgt] -> Gain5/1
  Gain4/1 -> [kinSw_alpha_start]
  Gain5/1 -> [kinSw_alpha_tgt]
  [tune_kinSw_gH_tgt] -> [kinSw_gH_tgt]
  [tune_kinSw_gClr_tgt] -> [kinSw_gClr_tgt]
  [poser_RLegAlp] -> Gain3/1
  [poser_LLegAlp] -> Gain2/1
  Gain2/1 -> Sum1/1
  Gain3/1 -> Sum/1
  Constant24/1 -> Sum/2, Sum1/2
  Constant1/1 -> Mux/1
  Constant3/1 -> Mux/2
  Constant4/1 -> Mux/3
  Constant5/1 -> Mux/4
  Constant7/1 -> Mux/5
  Constant8/1 -> Mux/6
  Gain/1 -> Mux/7
  Constant13/1 -> Mux/8
  Constant14/1 -> Mux/9
  Constant15/1 -> Mux/10
  Constant16/1 -> Mux/11
  [tune_M3_P] -> Mux/14, Mux/12
  [tune_M3_D] -> Mux/15, Mux/13
  Constant21/1 -> Mux/21, Mux/16
  Constant17/1 -> Mux/17
  Constant19/1 -> Mux/18
  Constant22/1 -> Mux/19
  Constant23/1 -> Mux/20
  Demux1/1 -> [tune_M1_G]
  Demux1/2 -> [tune_M3_0]
  Demux1/3 -> [tune_M3_P]
  Demux1/4 -> [tune_M3_D]
  Demux1/6 -> [tune_kinSw_alpha_start]
  Demux1/7 -> [tune_kinSw_alpha_tgt]
  Demux1/8 -> [tune_kinSw_gH_tgt]
  Demux1/9 -> [tune_kinSw_gClr_tgt]
  Demux1/12 -> [poser_LLegLen]
  Demux1/13 -> [poser_LLegAlp]
  Demux1/10 -> [poser_RLegLen]
  Demux1/11 -> [poser_RLegAlp]
  Demux1/5 -> [tune_M4_G]
  tunable inputs/1 -> Demux1/1
  [tune_M4_G] -> [M4_G]

== system atrias_boom_nmSt_kinSw_v4/Low Pass Discrete Derivative/discrete difference ==
  note: q Order:
      |
      | backJointR
      | backGearR
      | frontJointR
      | frontGearR
      |
      | backJointL
      | backGearL
      | frontJointL
      | frontGearL
      |
      | latR
      | latL
      |
      | boomRoll
      | boomYaw
      | boomPitch
  in : Inport
  Demux : Demux  Outputs=13
  Mux : Mux  Inputs=13
  difference : simulink/Discrete/Difference  ICPrevInput=shin_initial_r  InputProcessing=Columns as channels (frame based)  OutMin=[]  OutMax=[]  OutDataType=fixdt(1, 16)  OutScaling=2^-10  DoSatur=off
  difference1 : simulink/Discrete/Difference  ICPrevInput=shin_initial_r  InputProcessing=Columns as channels (frame based)  OutMin=[]  OutMax=[]  OutDataType=fixdt(1, 16)  OutScaling=2^-10  DoSatur=off
  difference10 : simulink/Discrete/Difference  ICPrevInput=initial_boom_roll  InputProcessing=Columns as channels (frame based)  OutMin=[]  OutMax=[]  OutDataType=fixdt(1, 16)  OutScaling=2^-10  DoSatur=off
  difference11 : simulink/Discrete/Difference  ICPrevInput=initial_boom_yaw  InputProcessing=Columns as channels (frame based)  OutMin=[]  OutMax=[]  OutDataType=fixdt(1, 16)  OutScaling=2^-10  DoSatur=off
  difference12 : simulink/Discrete/Difference  ICPrevInput=initial_boom_pitch  InputProcessing=Columns as channels (frame based)  OutMin=[]  OutMax=[]  OutDataType=fixdt(1, 16)  OutScaling=2^-10  DoSatur=off
  difference2 : simulink/Discrete/Difference  ICPrevInput=thigh_initial_r  InputProcessing=Columns as channels (frame based)  OutMin=[]  OutMax=[]  OutDataType=fixdt(1, 16)  OutScaling=2^-10  DoSatur=off
  difference3 : simulink/Discrete/Difference  ICPrevInput=thigh_initial_r  InputProcessing=Columns as channels (frame based)  OutMin=[]  OutMax=[]  OutDataType=fixdt(1, 16)  OutScaling=2^-10  DoSatur=off
  difference4 : simulink/Discrete/Difference  ICPrevInput=shin_initial_l  InputProcessing=Columns as channels (frame based)  OutMin=[]  OutMax=[]  OutDataType=fixdt(1, 16)  OutScaling=2^-10  DoSatur=off
  difference5 : simulink/Discrete/Difference  ICPrevInput=shin_initial_l  InputProcessing=Columns as channels (frame based)  OutMin=[]  OutMax=[]  OutDataType=fixdt(1, 16)  OutScaling=2^-10  DoSatur=off
  difference6 : simulink/Discrete/Difference  ICPrevInput=thigh_initial_l  InputProcessing=Columns as channels (frame based)  OutMin=[]  OutMax=[]  OutDataType=fixdt(1, 16)  OutScaling=2^-10  DoSatur=off
  difference7 : simulink/Discrete/Difference  ICPrevInput=thigh_initial_l  InputProcessing=Columns as channels (frame based)  OutMin=[]  OutMax=[]  OutDataType=fixdt(1, 16)  OutScaling=2^-10  DoSatur=off
  difference8 : simulink/Discrete/Difference  ICPrevInput=initial_hip_roll  InputProcessing=Columns as channels (frame based)  OutMin=[]  OutMax=[]  OutDataType=fixdt(1, 16)  OutScaling=2^-10  DoSatur=off
  difference9 : simulink/Discrete/Difference  ICPrevInput=initial_hip_roll  InputProcessing=Columns as channels (frame based)  OutMin=[]  OutMax=[]  OutDataType=fixdt(1, 16)  OutScaling=2^-10  DoSatur=off
  out : Outport
  wires:
  Demux/1 -> difference/1
  in/1 -> Demux/1
  Mux/1 -> out/1
  Demux/2 -> difference1/1
  difference1/1 -> Mux/2
  Demux/3 -> difference2/1
  difference2/1 -> Mux/3
  Demux/4 -> difference3/1
  difference3/1 -> Mux/4
  Demux/5 -> difference4/1
  difference4/1 -> Mux/5
  Demux/6 -> difference5/1
  difference5/1 -> Mux/6
  Demux/7 -> difference6/1
  difference6/1 -> Mux/7
  Demux/8 -> difference7/1
  difference7/1 -> Mux/8
  Demux/9 -> difference8/1
  difference8/1 -> Mux/9
  Demux/10 -> difference9/1
  difference9/1 -> Mux/10
  Demux/11 -> difference10/1
  difference10/1 -> Mux/11
  Demux/12 -> difference11/1
  difference11/1 -> Mux/12
  Demux/13 -> difference12/1
  difference12/1 -> Mux/13
  difference/1 -> Mux/1

== system atrias_boom_nmSt_kinSw_v4/Mechanical System Layer/Boom ==
  CS1 to CS2 : sm_lib/Frames and Transforms/Rigid Transform  TranslationMethod=Cartesian  TranslationLengthUnit=m  TranslationStandardAxis=+Z  TranslationStandardOffset=0  TranslationCartesianOffset=boom_12  TranslationROffset=0  TranslationROffsetUnits=m  TranslationZOffset=0  TranslationZOffsetUnits=m  TranslationThetaOffset=0  TranslationThetaOffsetUnits=deg  RotationMethod=None  RotationAngleUnits=deg  RotationStandardAxis=+Z  RotationAngle=0  RotationArbitraryAxis=[0 0 1]  FollAlignAxisA=+X  BaseAlignAxisA=+Y  FollAlignAxisB=+Y  BaseAlignAxisB=+Z  RotationMatrix=[1 0 0; 0 1 0; 0 0 1]  BlockFunction=simmechanics.library.frames_transforms.rigid_transform
  Frame Data : Subsystem
  Solid : sm_lib/Body Elements/Solid  InertiaType=Custom  Mass=m_boom  MassUnits=kg  CenterOfMass=com_boom  CenterOfMassUnits=m  MomentsOfInertia=i_boom_moments  MomentsOfInertiaUnits=kg*m^2  ProductsOfInertia=i_boom_products  ProductsOfInertiaUnits=kg*m^2  DensityBased=on  Density=1000  DensityUnits=kg/(m^3)  GraphicType=FromGeometry  MarkerShape=Sphere  MarkerSize=10  MarkerSizeUnits=m  GraphicVisPropType=AdvancedVisualProperties  GraphicDiffuseColor=boom_color_d  GraphicSpecularColor=[0.5 0.5 0.5 1.0]  GraphicAmbientColor=[boom_color_d*0.5 1.0]  GraphicEmissiveColor=[0.0 0.0 0.0 1.0]  GraphicShininess=128  GraphicOpacity=1.0  GeometryShape=FromFile  RectangleSize=[1 1]  RectangleSizeUnits=m  BrickDimensions=[1 1 1]  BrickDimensionUnits=m  CylinderRadius=l_rad  CylinderRadiusUnits=m  CylinderLength=l_seg  CylinderLengthUnits=m  SphereRadius=1  SphereRadiusUnits=m  EllipsoidRadii=[1 1 1]  EllipsoidRadiiUnits=m  ExtrusionCrossSection=[1 1; -1 1; -1 -1; 1 -1]  ExtrusionCrossSectionUnits=m  ExtrusionLength=1  ExtrusionLengthUnits=m  PolygonNumSides=3  PolygonOuterRadius=1  PolygonOuterRadiusUnits=m  ExtGeomFileType=STL  ExtGeomFileName=../models/boom_roll.stl  ExtGeomFileUnits=m  RevolutionCrossSection=[1 1; 1 -1; 2 -1; 2 1]  RevolutionCrossSectionUnits=m  RevolutionExtent=Full  RevolutionAngle=180  RevolutionAngleUnits=deg  BlockFunction=simmechanics.library.body_elements.solid
  CS1 : PMIOPort  Port=1  Side=Left
  CS2 : PMIOPort  Port=2  Side=Right
  connections:
  CS1/RConn1 -- Frame Data/LConn1 -- CS1 to CS2/LConn1 -- Solid/RConn1
  CS2/RConn1 -- CS1 to CS2/RConn1

== system atrias_boom_nmSt_kinSw_v4/Mechanical System Layer/Boom Base ==
  CS1 to CS2 : sm_lib/Frames and Transforms/Rigid Transform  TranslationMethod=Cartesian  TranslationLengthUnit=m  TranslationStandardAxis=+Z  TranslationStandardOffset=0  TranslationCartesianOffset=base_12  TranslationROffset=0  TranslationROffsetUnits=m  TranslationZOffset=0  TranslationZOffsetUnits=m  TranslationThetaOffset=0  TranslationThetaOffsetUnits=deg  RotationMethod=None  RotationAngleUnits=deg  RotationStandardAxis=+Z  RotationAngle=0  RotationArbitraryAxis=[0 0 1]  FollAlignAxisA=+X  BaseAlignAxisA=+Y  FollAlignAxisB=+Y  BaseAlignAxisB=+Z  RotationMatrix=[1 0 0; 0 1 0; 0 0 1]  BlockFunction=simmechanics.library.frames_transforms.rigid_transform
  Solid : sm_lib/Body Elements/Solid  InertiaType=PointMass  Mass=0  MassUnits=kg  CenterOfMass=[0 0 0]  CenterOfMassUnits=m  MomentsOfInertia=[0 0 0]  MomentsOfInertiaUnits=kg*m^2  ProductsOfInertia=[0 0 0]  ProductsOfInertiaUnits=kg*m^2  DensityBased=on  Density=1000  DensityUnits=kg/(m^3)  GraphicType=FromGeometry  MarkerShape=Sphere  MarkerSize=10  MarkerSizeUnits=m  GraphicVisPropType=AdvancedVisualProperties  GraphicDiffuseColor=base_color_d  GraphicSpecularColor=[0.5 0.5 0.5 1.0]  GraphicAmbientColor=[base_color_d*0.5 1.0]  GraphicEmissiveColor=[0.0 0.0 0.0 1.0]  GraphicShininess=128  GraphicOpacity=1.0  GeometryShape=FromFile  RectangleSize=[1 1]  RectangleSizeUnits=m  BrickDimensions=[1 1 1]  BrickDimensionUnits=m  CylinderRadius=l_rad  CylinderRadiusUnits=m  CylinderLength=l_seg  CylinderLengthUnits=m  SphereRadius=1  SphereRadiusUnits=m  EllipsoidRadii=[1 1 1]  EllipsoidRadiiUnits=m  ExtrusionCrossSection=[1 1; -1 1; -1 -1; 1 -1]  ExtrusionCrossSectionUnits=m  ExtrusionLength=1  ExtrusionLengthUnits=m  PolygonNumSides=3  PolygonOuterRadius=1  PolygonOuterRadiusUnits=m  ExtGeomFileType=STL  ExtGeomFileName=../models/boom_base.stl  ExtGeomFileUnits=m  RevolutionCrossSection=[1 1; 1 -1; 2 -1; 2 1]  RevolutionCrossSectionUnits=m  RevolutionExtent=Full  RevolutionAngle=180  RevolutionAngleUnits=deg  BlockFunction=simmechanics.library.body_elements.solid
  CS1 : PMIOPort  Port=1  Side=Left
  CS2 : PMIOPort  Port=2  Side=Right
  connections:
  CS1 to CS2/LConn1 -- CS1/RConn1 -- Solid/RConn1
  CS2/RConn1 -- CS1 to CS2/RConn1
